simulink model "gm_max_frequency_index"  (R2020a)
settings: Solver=FixedStepDiscrete  StartTime=0.0  StopTime=1e-2  RelTol=1e-3
model workspace (MAT data in the model file):
  amplitud = 2047
  fft_length = 32
  samples_per_period = 3
  sampling_time = 1e-06
libraries: simulink x384, dspsrcs4 x1, dsphdlxfrm x1, dspstat3 x1, hdlsllib x1
(part 15 of 18)

== system gm_max_frequency_index/max_index_frequency/frequency_max/index_finder/for_each_instance30/Iteration6 ==
  xin : Inport  OutDataTypeStr=fixdt(1, 13, 0)  SampleTime=3.2e-05
  yin : Inport  Port=2  OutDataTypeStr=fixdt(1, 13, 0)  SampleTime=3.2e-05
  idx : Inport  Port=3  OutDataTypeStr=fixdt(0, 5, 0)  SampleTime=3.2e-05
  MuxX : Switch  Criteria=u2 ~= 0  Threshold=double(0)  OutDataTypeStr=fixdt(1, 13, 0)  SampleTime=3.2e-05
  MuxY : Switch  Criteria=u2 ~= 0  Threshold=double(0)  OutDataTypeStr=fixdt(1, 13, 0)  SampleTime=3.2e-05
  XAdder : Sum  OutDataTypeStr=fixdt(1, 13, 0)  SampleTime=3.2e-05
  XSubtractor : Sum  Inputs=+-  AccumDataTypeStr=fixdt(1, 13, 0)  OutDataTypeStr=fixdt(1, 13, 0)  SampleTime=3.2e-05
  YAdder : Sum  OutDataTypeStr=fixdt(1, 13, 0)  SampleTime=3.2e-05
  YSub : Sum  Inputs=+-  AccumDataTypeStr=fixdt(1, 13, 0)  OutDataTypeStr=fixdt(1, 13, 0)  SampleTime=3.2e-05
  compare : simulink/Logic and Bit Operations/Compare To Constant  relop=<  const=double(0)  OutDataTypeStr=boolean
  dynamic_shift : ArithShift  BitShiftNumberSource=Input port  BitShiftDirection=Right
      settings: InputPortMap=u0,p1
  dynamic_shift1 : ArithShift  BitShiftNumberSource=Input port  BitShiftDirection=Right
      settings: InputPortMap=u0,p1
  xout : Outport  OutDataTypeStr=fixdt(1, 13, 0)
  yout : Outport  Port=2  OutDataTypeStr=fixdt(1, 13, 0)
  wires:
  idx/1 -> dynamic_shift1/2, dynamic_shift/2
  yin/1 -> YSub/1, YAdder/1, dynamic_shift1/1, compare/1
  xin/1 -> XAdder/1, XSubtractor/1, dynamic_shift/1
  YSub/1 -> MuxY/3
  YAdder/1 -> MuxY/1
  XAdder/1 -> MuxX/3
  XSubtractor/1 -> MuxX/1
  compare/1 -> MuxY/2, MuxX/2
  dynamic_shift1/1 -> XAdder/2, XSubtractor/2
  dynamic_shift/1 -> YSub/2, YAdder/2
  MuxY/1 -> yout/1
  MuxX/1 -> xout/1

== system gm_max_frequency_index/max_index_frequency/frequency_max/index_finder/for_each_instance30/Iteration7 ==
  xin : Inport  OutDataTypeStr=fixdt(1, 13, 0)  SampleTime=3.2e-05
  yin : Inport  Port=2  OutDataTypeStr=fixdt(1, 13, 0)  SampleTime=3.2e-05
  idx : Inport  Port=3  OutDataTypeStr=fixdt(0, 5, 0)  SampleTime=3.2e-05
  MuxX : Switch  Criteria=u2 ~= 0  Threshold=double(0)  OutDataTypeStr=fixdt(1, 13, 0)  SampleTime=3.2e-05
  MuxY : Switch  Criteria=u2 ~= 0  Threshold=double(0)  OutDataTypeStr=fixdt(1, 13, 0)  SampleTime=3.2e-05
  XAdder : Sum  OutDataTypeStr=fixdt(1, 13, 0)  SampleTime=3.2e-05
  XSubtractor : Sum  Inputs=+-  AccumDataTypeStr=fixdt(1, 13, 0)  OutDataTypeStr=fixdt(1, 13, 0)  SampleTime=3.2e-05
  YAdder : Sum  OutDataTypeStr=fixdt(1, 13, 0)  SampleTime=3.2e-05
  YSub : Sum  Inputs=+-  AccumDataTypeStr=fixdt(1, 13, 0)  OutDataTypeStr=fixdt(1, 13, 0)  SampleTime=3.2e-05
  compare : simulink/Logic and Bit Operations/Compare To Constant  relop=<  const=double(0)  OutDataTypeStr=boolean
  dynamic_shift : ArithShift  BitShiftNumberSource=Input port  BitShiftDirection=Right
      settings: InputPortMap=u0,p1
  dynamic_shift1 : ArithShift  BitShiftNumberSource=Input port  BitShiftDirection=Right
      settings: InputPortMap=u0,p1
  xout : Outport  OutDataTypeStr=fixdt(1, 13, 0)
  yout : Outport  Port=2  OutDataTypeStr=fixdt(1, 13, 0)
  wires:
  idx/1 -> dynamic_shift1/2, dynamic_shift/2
  yin/1 -> YSub/1, YAdder/1, dynamic_shift1/1, compare/1
  xin/1 -> XAdder/1, XSubtractor/1, dynamic_shift/1
  YSub/1 -> MuxY/3
  YAdder/1 -> MuxY/1
  XAdder/1 -> MuxX/3
  XSubtractor/1 -> MuxX/1
  compare/1 -> MuxY/2, MuxX/2
  dynamic_shift1/1 -> XAdder/2, XSubtractor/2
  dynamic_shift/1 -> YSub/2, YAdder/2
  MuxY/1 -> yout/1
  MuxX/1 -> xout/1

== system gm_max_frequency_index/max_index_frequency/frequency_max/index_finder/for_each_instance30/Iteration8 ==
  xin : Inport  OutDataTypeStr=fixdt(1, 13, 0)  SampleTime=3.2e-05
  yin : Inport  Port=2  OutDataTypeStr=fixdt(1, 13, 0)  SampleTime=3.2e-05
  idx : Inport  Port=3  OutDataTypeStr=fixdt(0, 5, 0)  SampleTime=3.2e-05
  MuxX : Switch  Criteria=u2 ~= 0  Threshold=double(0)  OutDataTypeStr=fixdt(1, 13, 0)  SampleTime=3.2e-05
  MuxY : Switch  Criteria=u2 ~= 0  Threshold=double(0)  OutDataTypeStr=fixdt(1, 13, 0)  SampleTime=3.2e-05
  XAdder : Sum  OutDataTypeStr=fixdt(1, 13, 0)  SampleTime=3.2e-05
  XSubtractor : Sum  Inputs=+-  AccumDataTypeStr=fixdt(1, 13, 0)  OutDataTypeStr=fixdt(1, 13, 0)  SampleTime=3.2e-05
  YAdder : Sum  OutDataTypeStr=fixdt(1, 13, 0)  SampleTime=3.2e-05
  YSub : Sum  Inputs=+-  AccumDataTypeStr=fixdt(1, 13, 0)  OutDataTypeStr=fixdt(1, 13, 0)  SampleTime=3.2e-05
  compare : simulink/Logic and Bit Operations/Compare To Constant  relop=<  const=double(0)  OutDataTypeStr=boolean
  dynamic_shift : ArithShift  BitShiftNumberSource=Input port  BitShiftDirection=Right
      settings: InputPortMap=u0,p1
  dynamic_shift1 : ArithShift  BitShiftNumberSource=Input port  BitShiftDirection=Right
      settings: InputPortMap=u0,p1
  xout : Outport  OutDataTypeStr=fixdt(1, 13, 0)
  yout : Outport  Port=2  OutDataTypeStr=fixdt(1, 13, 0)
  wires:
  idx/1 -> dynamic_shift1/2, dynamic_shift/2
  yin/1 -> YSub/1, YAdder/1, dynamic_shift1/1, compare/1
  xin/1 -> XAdder/1, XSubtractor/1, dynamic_shift/1
  YSub/1 -> MuxY/3
  YAdder/1 -> MuxY/1
  XAdder/1 -> MuxX/3
  XSubtractor/1 -> MuxX/1
  compare/1 -> MuxY/2, MuxX/2
  dynamic_shift1/1 -> XAdder/2, XSubtractor/2
  dynamic_shift/1 -> YSub/2, YAdder/2
  MuxY/1 -> yout/1
  MuxX/1 -> xout/1

== system gm_max_frequency_index/max_index_frequency/frequency_max/index_finder/for_each_instance30/Iteration9 ==
  xin : Inport  OutDataTypeStr=fixdt(1, 13, 0)  SampleTime=3.2e-05
  yin : Inport  Port=2  OutDataTypeStr=fixdt(1, 13, 0)  SampleTime=3.2e-05
  idx : Inport  Port=3  OutDataTypeStr=fixdt(0, 5, 0)  SampleTime=3.2e-05
  MuxX : Switch  Criteria=u2 ~= 0  Threshold=double(0)  OutDataTypeStr=fixdt(1, 13, 0)  SampleTime=3.2e-05
  MuxY : Switch  Criteria=u2 ~= 0  Threshold=double(0)  OutDataTypeStr=fixdt(1, 13, 0)  SampleTime=3.2e-05
  XAdder : Sum  OutDataTypeStr=fixdt(1, 13, 0)  SampleTime=3.2e-05
  XSubtractor : Sum  Inputs=+-  AccumDataTypeStr=fixdt(1, 13, 0)  OutDataTypeStr=fixdt(1, 13, 0)  SampleTime=3.2e-05
  YAdder : Sum  OutDataTypeStr=fixdt(1, 13, 0)  SampleTime=3.2e-05
  YSub : Sum  Inputs=+-  AccumDataTypeStr=fixdt(1, 13, 0)  OutDataTypeStr=fixdt(1, 13, 0)  SampleTime=3.2e-05
  compare : simulink/Logic and Bit Operations/Compare To Constant  relop=<  const=double(0)  OutDataTypeStr=boolean
  dynamic_shift : ArithShift  BitShiftNumberSource=Input port  BitShiftDirection=Right
      settings: InputPortMap=u0,p1
  dynamic_shift1 : ArithShift  BitShiftNumberSource=Input port  BitShiftDirection=Right
      settings: InputPortMap=u0,p1
  xout : Outport  OutDataTypeStr=fixdt(1, 13, 0)
  yout : Outport  Port=2  OutDataTypeStr=fixdt(1, 13, 0)
  wires:
  idx/1 -> dynamic_shift1/2, dynamic_shift/2
  yin/1 -> YSub/1, YAdder/1, dynamic_shift1/1, compare/1
  xin/1 -> XAdder/1, XSubtractor/1, dynamic_shift/1
  YSub/1 -> MuxY/3
  YAdder/1 -> MuxY/1
  XAdder/1 -> MuxX/3
  XSubtractor/1 -> MuxX/1
  compare/1 -> MuxY/2, MuxX/2
  dynamic_shift1/1 -> XAdder/2, XSubtractor/2
  dynamic_shift/1 -> YSub/2, YAdder/2
  MuxY/1 -> yout/1
  MuxX/1 -> xout/1

== system gm_max_frequency_index/max_index_frequency/frequency_max/index_finder/for_each_instance30/QuadrantMapper ==
  xin : Inport  OutDataTypeStr=fixdt(1, 13, 0)  SampleTime=3.2e-05
  yin : Inport  Port=2  OutDataTypeStr=fixdt(1, 13, 0)  SampleTime=3.2e-05
  abs : Abs  SampleTime=3.2e-05  OutDataTypeStr=fixdt(1, 13, 0)
  abs1 : Abs  SampleTime=3.2e-05  OutDataTypeStr=fixdt(1, 13, 0)
  delayMatch{,1..3} (4 alike) : Delay  DelayLength=double(1)  InitialCondition=0  SampleTime=3.2e-05
  mux : MultiPortSwitch  DataPortOrder=Zero-based contiguous  Inputs=2  DiagnosticForDefault=None  zeroidx=on  OutDataTypeStr=fixdt(1, 13, 0)  SampleTime=3.2e-05
  mux1 : MultiPortSwitch  DataPortOrder=Zero-based contiguous  Inputs=2  DiagnosticForDefault=None  zeroidx=on  OutDataTypeStr=fixdt(1, 13, 0)  SampleTime=3.2e-05
  relop : RelationalOperator  Operator=>  OutDataTypeStr=fixdt(0, 1, 0)  SampleTime=3.2e-05  RndMeth=Nearest  InputSameDT=on
  xout : Outport  OutDataTypeStr=fixdt(1, 13, 0)
  yout : Outport  Port=2  OutDataTypeStr=fixdt(1, 13, 0)
  wires:
  relop/1 -> mux1/1, mux/1
  mux1/1 -> delayMatch3/1
  mux/1 -> delayMatch2/1
  abs1/1 -> delayMatch1/1
  abs/1 -> delayMatch/1
  yin/1 -> abs1/1
  xin/1 -> abs/1
  delayMatch1/1 -> mux/3, mux1/2, relop/2
  delayMatch/1 -> mux/2, mux1/3, relop/1
  delayMatch2/1 -> yout/1
  delayMatch3/1 -> xout/1

== system gm_max_frequency_index/max_index_frequency/frequency_max/index_finder/for_each_instance31/Iteration ==
  xin : Inport  OutDataTypeStr=fixdt(1, 13, 0)  SampleTime=3.2e-05
  yin : Inport  Port=2  OutDataTypeStr=fixdt(1, 13, 0)  SampleTime=3.2e-05
  idx : Inport  Port=3  OutDataTypeStr=fixdt(0, 5, 0)  SampleTime=3.2e-05
  MuxX : Switch  Criteria=u2 ~= 0  Threshold=double(0)  OutDataTypeStr=fixdt(1, 13, 0)  SampleTime=3.2e-05
  MuxY : Switch  Criteria=u2 ~= 0  Threshold=double(0)  OutDataTypeStr=fixdt(1, 13, 0)  SampleTime=3.2e-05
  XAdder : Sum  OutDataTypeStr=fixdt(1, 13, 0)  SampleTime=3.2e-05
  XSubtractor : Sum  Inputs=+-  AccumDataTypeStr=fixdt(1, 13, 0)  OutDataTypeStr=fixdt(1, 13, 0)  SampleTime=3.2e-05
  YAdder : Sum  OutDataTypeStr=fixdt(1, 13, 0)  SampleTime=3.2e-05
  YSub : Sum  Inputs=+-  AccumDataTypeStr=fixdt(1, 13, 0)  OutDataTypeStr=fixdt(1, 13, 0)  SampleTime=3.2e-05
  compare : simulink/Logic and Bit Operations/Compare To Constant  relop=<  const=double(0)  OutDataTypeStr=boolean
  dynamic_shift : ArithShift  BitShiftNumberSource=Input port  BitShiftDirection=Right
      settings: InputPortMap=u0,p1
  dynamic_shift1 : ArithShift  BitShiftNumberSource=Input port  BitShiftDirection=Right
      settings: InputPortMap=u0,p1
  xout : Outport  OutDataTypeStr=fixdt(1, 13, 0)
  yout : Outport  Port=2  OutDataTypeStr=fixdt(1, 13, 0)
  wires:
  idx/1 -> dynamic_shift1/2, dynamic_shift/2
  yin/1 -> YSub/1, YAdder/1, dynamic_shift1/1, compare/1
  xin/1 -> XAdder/1, XSubtractor/1, dynamic_shift/1
  YSub/1 -> MuxY/3
  YAdder/1 -> MuxY/1
  XAdder/1 -> MuxX/3
  XSubtractor/1 -> MuxX/1
  compare/1 -> MuxY/2, MuxX/2
  dynamic_shift1/1 -> XAdder/2, XSubtractor/2
  dynamic_shift/1 -> YSub/2, YAdder/2
  MuxY/1 -> yout/1
  MuxX/1 -> xout/1

== system gm_max_frequency_index/max_index_frequency/frequency_max/index_finder/for_each_instance31/Iteration1 ==
  xin : Inport  OutDataTypeStr=fixdt(1, 13, 0)  SampleTime=3.2e-05
  yin : Inport  Port=2  OutDataTypeStr=fixdt(1, 13, 0)  SampleTime=3.2e-05
  idx : Inport  Port=3  OutDataTypeStr=fixdt(0, 5, 0)  SampleTime=3.2e-05
  MuxX : Switch  Criteria=u2 ~= 0  Threshold=double(0)  OutDataTypeStr=fixdt(1, 13, 0)  SampleTime=3.2e-05
  MuxY : Switch  Criteria=u2 ~= 0  Threshold=double(0)  OutDataTypeStr=fixdt(1, 13, 0)  SampleTime=3.2e-05
  XAdder : Sum  OutDataTypeStr=fixdt(1, 13, 0)  SampleTime=3.2e-05
  XSubtractor : Sum  Inputs=+-  AccumDataTypeStr=fixdt(1, 13, 0)  OutDataTypeStr=fixdt(1, 13, 0)  SampleTime=3.2e-05
  YAdder : Sum  OutDataTypeStr=fixdt(1, 13, 0)  SampleTime=3.2e-05
  YSub : Sum  Inputs=+-  AccumDataTypeStr=fixdt(1, 13, 0)  OutDataTypeStr=fixdt(1, 13, 0)  SampleTime=3.2e-05
  compare : simulink/Logic and Bit Operations/Compare To Constant  relop=<  const=double(0)  OutDataTypeStr=boolean
  dynamic_shift : ArithShift  BitShiftNumberSource=Input port  BitShiftDirection=Right
      settings: InputPortMap=u0,p1
  dynamic_shift1 : ArithShift  BitShiftNumberSource=Input port  BitShiftDirection=Right
      settings: InputPortMap=u0,p1
  xout : Outport  OutDataTypeStr=fixdt(1, 13, 0)
  yout : Outport  Port=2  OutDataTypeStr=fixdt(1, 13, 0)
  wires:
  idx/1 -> dynamic_shift1/2, dynamic_shift/2
  yin/1 -> YSub/1, YAdder/1, dynamic_shift1/1, compare/1
  xin/1 -> XAdder/1, XSubtractor/1, dynamic_shift/1
  YSub/1 -> MuxY/3
  YAdder/1 -> MuxY/1
  XAdder/1 -> MuxX/3
  XSubtractor/1 -> MuxX/1
  compare/1 -> MuxY/2, MuxX/2
  dynamic_shift1/1 -> XAdder/2, XSubtractor/2
  dynamic_shift/1 -> YSub/2, YAdder/2
  MuxY/1 -> yout/1
  MuxX/1 -> xout/1

== system gm_max_frequency_index/max_index_frequency/frequency_max/index_finder/for_each_instance31/Iteration10 ==
  xin : Inport  OutDataTypeStr=fixdt(1, 13, 0)  SampleTime=3.2e-05
  yin : Inport  Port=2  OutDataTypeStr=fixdt(1, 13, 0)  SampleTime=3.2e-05
  idx : Inport  Port=3  OutDataTypeStr=fixdt(0, 5, 0)  SampleTime=3.2e-05
  MuxX : Switch  Criteria=u2 ~= 0  Threshold=double(0)  OutDataTypeStr=fixdt(1, 13, 0)  SampleTime=3.2e-05
  MuxY : Switch  Criteria=u2 ~= 0  Threshold=double(0)  OutDataTypeStr=fixdt(1, 13, 0)  SampleTime=3.2e-05
  XAdder : Sum  OutDataTypeStr=fixdt(1, 13, 0)  SampleTime=3.2e-05
  XSubtractor : Sum  Inputs=+-  AccumDataTypeStr=fixdt(1, 13, 0)  OutDataTypeStr=fixdt(1, 13, 0)  SampleTime=3.2e-05
  YAdder : Sum  OutDataTypeStr=fixdt(1, 13, 0)  SampleTime=3.2e-05
  YSub : Sum  Inputs=+-  AccumDataTypeStr=fixdt(1, 13, 0)  OutDataTypeStr=fixdt(1, 13, 0)  SampleTime=3.2e-05
  compare : simulink/Logic and Bit Operations/Compare To Constant  relop=<  const=double(0)  OutDataTypeStr=boolean
  dynamic_shift : ArithShift  BitShiftNumberSource=Input port  BitShiftDirection=Right
      settings: InputPortMap=u0,p1
  dynamic_shift1 : ArithShift  BitShiftNumberSource=Input port  BitShiftDirection=Right
      settings: InputPortMap=u0,p1
  xout : Outport  OutDataTypeStr=fixdt(1, 13, 0)
  yout : Outport  Port=2  OutDataTypeStr=fixdt(1, 13, 0)
  wires:
  idx/1 -> dynamic_shift/2, dynamic_shift1/2
  yin/1 -> compare/1, dynamic_shift1/1, YAdder/1, YSub/1
  xin/1 -> dynamic_shift/1, XSubtractor/1, XAdder/1
  YSub/1 -> MuxY/3
  YAdder/1 -> MuxY/1
  XAdder/1 -> MuxX/3
  XSubtractor/1 -> MuxX/1
  compare/1 -> MuxX/2, MuxY/2
  dynamic_shift1/1 -> XSubtractor/2, XAdder/2
  dynamic_shift/1 -> YAdder/2, YSub/2
  MuxY/1 -> yout/1
  MuxX/1 -> xout/1

== system gm_max_frequency_index/max_index_frequency/frequency_max/index_finder/for_each_instance31/Iteration2 ==
  xin : Inport  OutDataTypeStr=fixdt(1, 13, 0)  SampleTime=3.2e-05
  yin : Inport  Port=2  OutDataTypeStr=fixdt(1, 13, 0)  SampleTime=3.2e-05
  idx : Inport  Port=3  OutDataTypeStr=fixdt(0, 5, 0)  SampleTime=3.2e-05
  MuxX : Switch  Criteria=u2 ~= 0  Threshold=double(0)  OutDataTypeStr=fixdt(1, 13, 0)  SampleTime=3.2e-05
  MuxY : Switch  Criteria=u2 ~= 0  Threshold=double(0)  OutDataTypeStr=fixdt(1, 13, 0)  SampleTime=3.2e-05
  XAdder : Sum  OutDataTypeStr=fixdt(1, 13, 0)  SampleTime=3.2e-05
  XSubtractor : Sum  Inputs=+-  AccumDataTypeStr=fixdt(1, 13, 0)  OutDataTypeStr=fixdt(1, 13, 0)  SampleTime=3.2e-05
  YAdder : Sum  OutDataTypeStr=fixdt(1, 13, 0)  SampleTime=3.2e-05
  YSub : Sum  Inputs=+-  AccumDataTypeStr=fixdt(1, 13, 0)  OutDataTypeStr=fixdt(1, 13, 0)  SampleTime=3.2e-05
  compare : simulink/Logic and Bit Operations/Compare To Constant  relop=<  const=double(0)  OutDataTypeStr=boolean
  dynamic_shift : ArithShift  BitShiftNumberSource=Input port  BitShiftDirection=Right
      settings: InputPortMap=u0,p1
  dynamic_shift1 : ArithShift  BitShiftNumberSource=Input port  BitShiftDirection=Right
      settings: InputPortMap=u0,p1
  xout : Outport  OutDataTypeStr=fixdt(1, 13, 0)
  yout : Outport  Port=2  OutDataTypeStr=fixdt(1, 13, 0)
  wires:
  idx/1 -> dynamic_shift1/2, dynamic_shift/2
  yin/1 -> YSub/1, YAdder/1, dynamic_shift1/1, compare/1
  xin/1 -> XAdder/1, XSubtractor/1, dynamic_shift/1
  YSub/1 -> MuxY/3
  YAdder/1 -> MuxY/1
  XAdder/1 -> MuxX/3
  XSubtractor/1 -> MuxX/1
  compare/1 -> MuxY/2, MuxX/2
  dynamic_shift1/1 -> XAdder/2, XSubtractor/2
  dynamic_shift/1 -> YSub/2, YAdder/2
  MuxY/1 -> yout/1
  MuxX/1 -> xout/1

== system gm_max_frequency_index/max_index_frequency/frequency_max/index_finder/for_each_instance31/Iteration3 ==
  xin : Inport  OutDataTypeStr=fixdt(1, 13, 0)  SampleTime=3.2e-05
  yin : Inport  Port=2  OutDataTypeStr=fixdt(1, 13, 0)  SampleTime=3.2e-05
  idx : Inport  Port=3  OutDataTypeStr=fixdt(0, 5, 0)  SampleTime=3.2e-05
  MuxX : Switch  Criteria=u2 ~= 0  Threshold=double(0)  OutDataTypeStr=fixdt(1, 13, 0)  SampleTime=3.2e-05
  MuxY : Switch  Criteria=u2 ~= 0  Threshold=double(0)  OutDataTypeStr=fixdt(1, 13, 0)  SampleTime=3.2e-05
  XAdder : Sum  OutDataTypeStr=fixdt(1, 13, 0)  SampleTime=3.2e-05
  XSubtractor : Sum  Inputs=+-  AccumDataTypeStr=fixdt(1, 13, 0)  OutDataTypeStr=fixdt(1, 13, 0)  SampleTime=3.2e-05
  YAdder : Sum  OutDataTypeStr=fixdt(1, 13, 0)  SampleTime=3.2e-05
  YSub : Sum  Inputs=+-  AccumDataTypeStr=fixdt(1, 13, 0)  OutDataTypeStr=fixdt(1, 13, 0)  SampleTime=3.2e-05
  compare : simulink/Logic and Bit Operations/Compare To Constant  relop=<  const=double(0)  OutDataTypeStr=boolean
  dynamic_shift : ArithShift  BitShiftNumberSource=Input port  BitShiftDirection=Right
      settings: InputPortMap=u0,p1
  dynamic_shift1 : ArithShift  BitShiftNumberSource=Input port  BitShiftDirection=Right
      settings: InputPortMap=u0,p1
  xout : Outport  OutDataTypeStr=fixdt(1, 13, 0)
  yout : Outport  Port=2  OutDataTypeStr=fixdt(1, 13, 0)
  wires:
  idx/1 -> dynamic_shift1/2, dynamic_shift/2
  yin/1 -> YSub/1, YAdder/1, dynamic_shift1/1, compare/1
  xin/1 -> XAdder/1, XSubtractor/1, dynamic_shift/1
  YSub/1 -> MuxY/3
  YAdder/1 -> MuxY/1
  XAdder/1 -> MuxX/3
  XSubtractor/1 -> MuxX/1
  compare/1 -> MuxY/2, MuxX/2
  dynamic_shift1/1 -> XAdder/2, XSubtractor/2
  dynamic_shift/1 -> YSub/2, YAdder/2
  MuxY/1 -> yout/1
  MuxX/1 -> xout/1

== system gm_max_frequency_index/max_index_frequency/frequency_max/index_finder/for_each_instance31/Iteration4 ==
  xin : Inport  OutDataTypeStr=fixdt(1, 13, 0)  SampleTime=3.2e-05
  yin : Inport  Port=2  OutDataTypeStr=fixdt(1, 13, 0)  SampleTime=3.2e-05
  idx : Inport  Port=3  OutDataTypeStr=fixdt(0, 5, 0)  SampleTime=3.2e-05
  MuxX : Switch  Criteria=u2 ~= 0  Threshold=double(0)  OutDataTypeStr=fixdt(1, 13, 0)  SampleTime=3.2e-05
  MuxY : Switch  Criteria=u2 ~= 0  Threshold=double(0)  OutDataTypeStr=fixdt(1, 13, 0)  SampleTime=3.2e-05
  XAdder : Sum  OutDataTypeStr=fixdt(1, 13, 0)  SampleTime=3.2e-05
  XSubtractor : Sum  Inputs=+-  AccumDataTypeStr=fixdt(1, 13, 0)  OutDataTypeStr=fixdt(1, 13, 0)  SampleTime=3.2e-05
  YAdder : Sum  OutDataTypeStr=fixdt(1, 13, 0)  SampleTime=3.2e-05
  YSub : Sum  Inputs=+-  AccumDataTypeStr=fixdt(1, 13, 0)  OutDataTypeStr=fixdt(1, 13, 0)  SampleTime=3.2e-05
  compare : simulink/Logic and Bit Operations/Compare To Constant  relop=<  const=double(0)  OutDataTypeStr=boolean
  dynamic_shift : ArithShift  BitShiftNumberSource=Input port  BitShiftDirection=Right
      settings: InputPortMap=u0,p1
  dynamic_shift1 : ArithShift  BitShiftNumberSource=Input port  BitShiftDirection=Right
      settings: InputPortMap=u0,p1
  xout : Outport  OutDataTypeStr=fixdt(1, 13, 0)
  yout : Outport  Port=2  OutDataTypeStr=fixdt(1, 13, 0)
  wires:
  idx/1 -> dynamic_shift1/2, dynamic_shift/2
  yin/1 -> YSub/1, YAdder/1, dynamic_shift1/1, compare/1
  xin/1 -> XAdder/1, XSubtractor/1, dynamic_shift/1
  YSub/1 -> MuxY/3
  YAdder/1 -> MuxY/1
  XAdder/1 -> MuxX/3
  XSubtractor/1 -> MuxX/1
  compare/1 -> MuxY/2, MuxX/2
  dynamic_shift1/1 -> XAdder/2, XSubtractor/2
  dynamic_shift/1 -> YSub/2, YAdder/2
  MuxY/1 -> yout/1
  MuxX/1 -> xout/1

== system gm_max_frequency_index/max_index_frequency/frequency_max/index_finder/for_each_instance31/Iteration5 ==
  xin : Inport  OutDataTypeStr=fixdt(1, 13, 0)  SampleTime=3.2e-05
  yin : Inport  Port=2  OutDataTypeStr=fixdt(1, 13, 0)  SampleTime=3.2e-05
  idx : Inport  Port=3  OutDataTypeStr=fixdt(0, 5, 0)  SampleTime=3.2e-05
  MuxX : Switch  Criteria=u2 ~= 0  Threshold=double(0)  OutDataTypeStr=fixdt(1, 13, 0)  SampleTime=3.2e-05
  MuxY : Switch  Criteria=u2 ~= 0  Threshold=double(0)  OutDataTypeStr=fixdt(1, 13, 0)  SampleTime=3.2e-05
  XAdder : Sum  OutDataTypeStr=fixdt(1, 13, 0)  SampleTime=3.2e-05
  XSubtractor : Sum  Inputs=+-  AccumDataTypeStr=fixdt(1, 13, 0)  OutDataTypeStr=fixdt(1, 13, 0)  SampleTime=3.2e-05
  YAdder : Sum  OutDataTypeStr=fixdt(1, 13, 0)  SampleTime=3.2e-05
  YSub : Sum  Inputs=+-  AccumDataTypeStr=fixdt(1, 13, 0)  OutDataTypeStr=fixdt(1, 13, 0)  SampleTime=3.2e-05
  compare : simulink/Logic and Bit Operations/Compare To Constant  relop=<  const=double(0)  OutDataTypeStr=boolean
  dynamic_shift : ArithShift  BitShiftNumberSource=Input port  BitShiftDirection=Right
      settings: InputPortMap=u0,p1
  dynamic_shift1 : ArithShift  BitShiftNumberSource=Input port  BitShiftDirection=Right
      settings: InputPortMap=u0,p1
  xout : Outport  OutDataTypeStr=fixdt(1, 13, 0)
  yout : Outport  Port=2  OutDataTypeStr=fixdt(1, 13, 0)
  wires:
  idx/1 -> dynamic_shift1/2, dynamic_shift/2
  yin/1 -> YSub/1, YAdder/1, dynamic_shift1/1, compare/1
  xin/1 -> XAdder/1, XSubtractor/1, dynamic_shift/1
  YSub/1 -> MuxY/3
  YAdder/1 -> MuxY/1
  XAdder/1 -> MuxX/3
  XSubtractor/1 -> MuxX/1
  compare/1 -> MuxY/2, MuxX/2
  dynamic_shift1/1 -> XAdder/2, XSubtractor/2
  dynamic_shift/1 -> YSub/2, YAdder/2
  MuxY/1 -> yout/1
  MuxX/1 -> xout/1

== system gm_max_frequency_index/max_index_frequency/frequency_max/index_finder/for_each_instance31/Iteration6 ==
  xin : Inport  OutDataTypeStr=fixdt(1, 13, 0)  SampleTime=3.2e-05
  yin : Inport  Port=2  OutDataTypeStr=fixdt(1, 13, 0)  SampleTime=3.2e-05
  idx : Inport  Port=3  OutDataTypeStr=fixdt(0, 5, 0)  SampleTime=3.2e-05
  MuxX : Switch  Criteria=u2 ~= 0  Threshold=double(0)  OutDataTypeStr=fixdt(1, 13, 0)  SampleTime=3.2e-05
  MuxY : Switch  Criteria=u2 ~= 0  Threshold=double(0)  OutDataTypeStr=fixdt(1, 13, 0)  SampleTime=3.2e-05
  XAdder : Sum  OutDataTypeStr=fixdt(1, 13, 0)  SampleTime=3.2e-05
  XSubtractor : Sum  Inputs=+-  AccumDataTypeStr=fixdt(1, 13, 0)  OutDataTypeStr=fixdt(1, 13, 0)  SampleTime=3.2e-05
  YAdder : Sum  OutDataTypeStr=fixdt(1, 13, 0)  SampleTime=3.2e-05
  YSub : Sum  Inputs=+-  AccumDataTypeStr=fixdt(1, 13, 0)  OutDataTypeStr=fixdt(1, 13, 0)  SampleTime=3.2e-05
  compare : simulink/Logic and Bit Operations/Compare To Constant  relop=<  const=double(0)  OutDataTypeStr=boolean
  dynamic_shift : ArithShift  BitShiftNumberSource=Input port  BitShiftDirection=Right
      settings: InputPortMap=u0,p1
  dynamic_shift1 : ArithShift  BitShiftNumberSource=Input port  BitShiftDirection=Right
      settings: InputPortMap=u0,p1
  xout : Outport  OutDataTypeStr=fixdt(1, 13, 0)
  yout : Outport  Port=2  OutDataTypeStr=fixdt(1, 13, 0)
  wires:
  idx/1 -> dynamic_shift1/2, dynamic_shift/2
  yin/1 -> YSub/1, YAdder/1, dynamic_shift1/1, compare/1
  xin/1 -> XAdder/1, XSubtractor/1, dynamic_shift/1
  YSub/1 -> MuxY/3
  YAdder/1 -> MuxY/1
  XAdder/1 -> MuxX/3
  XSubtractor/1 -> MuxX/1
  compare/1 -> MuxY/2, MuxX/2
  dynamic_shift1/1 -> XAdder/2, XSubtractor/2
  dynamic_shift/1 -> YSub/2, YAdder/2
  MuxY/1 -> yout/1
  MuxX/1 -> xout/1

== system gm_max_frequency_index/max_index_frequency/frequency_max/index_finder/for_each_instance31/Iteration7 ==
  xin : Inport  OutDataTypeStr=fixdt(1, 13, 0)  SampleTime=3.2e-05
  yin : Inport  Port=2  OutDataTypeStr=fixdt(1, 13, 0)  SampleTime=3.2e-05
  idx : Inport  Port=3  OutDataTypeStr=fixdt(0, 5, 0)  SampleTime=3.2e-05
  MuxX : Switch  Criteria=u2 ~= 0  Threshold=double(0)  OutDataTypeStr=fixdt(1, 13, 0)  SampleTime=3.2e-05
  MuxY : Switch  Criteria=u2 ~= 0  Threshold=double(0)  OutDataTypeStr=fixdt(1, 13, 0)  SampleTime=3.2e-05
  XAdder : Sum  OutDataTypeStr=fixdt(1, 13, 0)  SampleTime=3.2e-05
  XSubtractor : Sum  Inputs=+-  AccumDataTypeStr=fixdt(1, 13, 0)  OutDataTypeStr=fixdt(1, 13, 0)  SampleTime=3.2e-05
  YAdder : Sum  OutDataTypeStr=fixdt(1, 13, 0)  SampleTime=3.2e-05
  YSub : Sum  Inputs=+-  AccumDataTypeStr=fixdt(1, 13, 0)  OutDataTypeStr=fixdt(1, 13, 0)  SampleTime=3.2e-05
  compare : simulink/Logic and Bit Operations/Compare To Constant  relop=<  const=double(0)  OutDataTypeStr=boolean
  dynamic_shift : ArithShift  BitShiftNumberSource=Input port  BitShiftDirection=Right
      settings: InputPortMap=u0,p1
  dynamic_shift1 : ArithShift  BitShiftNumberSource=Input port  BitShiftDirection=Right
      settings: InputPortMap=u0,p1
  xout : Outport  OutDataTypeStr=fixdt(1, 13, 0)
  yout : Outport  Port=2  OutDataTypeStr=fixdt(1, 13, 0)
  wires:
  idx/1 -> dynamic_shift1/2, dynamic_shift/2
  yin/1 -> YSub/1, YAdder/1, dynamic_shift1/1, compare/1
  xin/1 -> XAdder/1, XSubtractor/1, dynamic_shift/1
  YSub/1 -> MuxY/3
  YAdder/1 -> MuxY/1
  XAdder/1 -> MuxX/3
  XSubtractor/1 -> MuxX/1
  compare/1 -> MuxY/2, MuxX/2
  dynamic_shift1/1 -> XAdder/2, XSubtractor/2
  dynamic_shift/1 -> YSub/2, YAdder/2
  MuxY/1 -> yout/1
  MuxX/1 -> xout/1

== system gm_max_frequency_index/max_index_frequency/frequency_max/index_finder/for_each_instance31/Iteration8 ==
  xin : Inport  OutDataTypeStr=fixdt(1, 13, 0)  SampleTime=3.2e-05
  yin : Inport  Port=2  OutDataTypeStr=fixdt(1, 13, 0)  SampleTime=3.2e-05
  idx : Inport  Port=3  OutDataTypeStr=fixdt(0, 5, 0)  SampleTime=3.2e-05
  MuxX : Switch  Criteria=u2 ~= 0  Threshold=double(0)  OutDataTypeStr=fixdt(1, 13, 0)  SampleTime=3.2e-05
  MuxY : Switch  Criteria=u2 ~= 0  Threshold=double(0)  OutDataTypeStr=fixdt(1, 13, 0)  SampleTime=3.2e-05
  XAdder : Sum  OutDataTypeStr=fixdt(1, 13, 0)  SampleTime=3.2e-05
  XSubtractor : Sum  Inputs=+-  AccumDataTypeStr=fixdt(1, 13, 0)  OutDataTypeStr=fixdt(1, 13, 0)  SampleTime=3.2e-05
  YAdder : Sum  OutDataTypeStr=fixdt(1, 13, 0)  SampleTime=3.2e-05
  YSub : Sum  Inputs=+-  AccumDataTypeStr=fixdt(1, 13, 0)  OutDataTypeStr=fixdt(1, 13, 0)  SampleTime=3.2e-05
  compare : simulink/Logic and Bit Operations/Compare To Constant  relop=<  const=double(0)  OutDataTypeStr=boolean
  dynamic_shift : ArithShift  BitShiftNumberSource=Input port  BitShiftDirection=Right
      settings: InputPortMap=u0,p1
  dynamic_shift1 : ArithShift  BitShiftNumberSource=Input port  BitShiftDirection=Right
      settings: InputPortMap=u0,p1
  xout : Outport  OutDataTypeStr=fixdt(1, 13, 0)
  yout : Outport  Port=2  OutDataTypeStr=fixdt(1, 13, 0)
  wires:
  idx/1 -> dynamic_shift1/2, dynamic_shift/2
  yin/1 -> YSub/1, YAdder/1, dynamic_shift1/1, compare/1
  xin/1 -> XAdder/1, XSubtractor/1, dynamic_shift/1
  YSub/1 -> MuxY/3
  YAdder/1 -> MuxY/1
  XAdder/1 -> MuxX/3
  XSubtractor/1 -> MuxX/1
  compare/1 -> MuxY/2, MuxX/2
  dynamic_shift1/1 -> XAdder/2, XSubtractor/2
  dynamic_shift/1 -> YSub/2, YAdder/2
  MuxY/1 -> yout/1
  MuxX/1 -> xout/1

== system gm_max_frequency_index/max_index_frequency/frequency_max/index_finder/for_each_instance31/Iteration9 ==
  xin : Inport  OutDataTypeStr=fixdt(1, 13, 0)  SampleTime=3.2e-05
  yin : Inport  Port=2  OutDataTypeStr=fixdt(1, 13, 0)  SampleTime=3.2e-05
  idx : Inport  Port=3  OutDataTypeStr=fixdt(0, 5, 0)  SampleTime=3.2e-05
  MuxX : Switch  Criteria=u2 ~= 0  Threshold=double(0)  OutDataTypeStr=fixdt(1, 13, 0)  SampleTime=3.2e-05
  MuxY : Switch  Criteria=u2 ~= 0  Threshold=double(0)  OutDataTypeStr=fixdt(1, 13, 0)  SampleTime=3.2e-05
  XAdder : Sum  OutDataTypeStr=fixdt(1, 13, 0)  SampleTime=3.2e-05
  XSubtractor : Sum  Inputs=+-  AccumDataTypeStr=fixdt(1, 13, 0)  OutDataTypeStr=fixdt(1, 13, 0)  SampleTime=3.2e-05
  YAdder : Sum  OutDataTypeStr=fixdt(1, 13, 0)  SampleTime=3.2e-05
  YSub : Sum  Inputs=+-  AccumDataTypeStr=fixdt(1, 13, 0)  OutDataTypeStr=fixdt(1, 13, 0)  SampleTime=3.2e-05
  compare : simulink/Logic and Bit Operations/Compare To Constant  relop=<  const=double(0)  OutDataTypeStr=boolean
  dynamic_shift : ArithShift  BitShiftNumberSource=Input port  BitShiftDirection=Right
      settings: InputPortMap=u0,p1
  dynamic_shift1 : ArithShift  BitShiftNumberSource=Input port  BitShiftDirection=Right
      settings: InputPortMap=u0,p1
  xout : Outport  OutDataTypeStr=fixdt(1, 13, 0)
  yout : Outport  Port=2  OutDataTypeStr=fixdt(1, 13, 0)
  wires:
  idx/1 -> dynamic_shift1/2, dynamic_shift/2
  yin/1 -> YSub/1, YAdder/1, dynamic_shift1/1, compare/1
  xin/1 -> XAdder/1, XSubtractor/1, dynamic_shift/1
  YSub/1 -> MuxY/3
  YAdder/1 -> MuxY/1
  XAdder/1 -> MuxX/3
  XSubtractor/1 -> MuxX/1
  compare/1 -> MuxY/2, MuxX/2
  dynamic_shift1/1 -> XAdder/2, XSubtractor/2
  dynamic_shift/1 -> YSub/2, YAdder/2
  MuxY/1 -> yout/1
  MuxX/1 -> xout/1

== system gm_max_frequency_index/max_index_frequency/frequency_max/index_finder/for_each_instance31/QuadrantMapper ==
  xin : Inport  OutDataTypeStr=fixdt(1, 13, 0)  SampleTime=3.2e-05
  yin : Inport  Port=2  OutDataTypeStr=fixdt(1, 13, 0)  SampleTime=3.2e-05
  abs : Abs  SampleTime=3.2e-05  OutDataTypeStr=fixdt(1, 13, 0)
  abs1 : Abs  SampleTime=3.2e-05  OutDataTypeStr=fixdt(1, 13, 0)
  delayMatch{,1..3} (4 alike) : Delay  DelayLength=double(1)  InitialCondition=0  SampleTime=3.2e-05
  mux : MultiPortSwitch  DataPortOrder=Zero-based contiguous  Inputs=2  DiagnosticForDefault=None  zeroidx=on  OutDataTypeStr=fixdt(1, 13, 0)  SampleTime=3.2e-05
  mux1 : MultiPortSwitch  DataPortOrder=Zero-based contiguous  Inputs=2  DiagnosticForDefault=None  zeroidx=on  OutDataTypeStr=fixdt(1, 13, 0)  SampleTime=3.2e-05
  relop : RelationalOperator  Operator=>  OutDataTypeStr=fixdt(0, 1, 0)  SampleTime=3.2e-05  RndMeth=Nearest  InputSameDT=on
  xout : Outport  OutDataTypeStr=fixdt(1, 13, 0)
  yout : Outport  Port=2  OutDataTypeStr=fixdt(1, 13, 0)
  wires:
  relop/1 -> mux1/1, mux/1
  mux1/1 -> delayMatch3/1
  mux/1 -> delayMatch2/1
  abs1/1 -> delayMatch1/1
  abs/1 -> delayMatch/1
  yin/1 -> abs1/1
  xin/1 -> abs/1
  delayMatch1/1 -> mux/3, mux1/2, relop/2
  delayMatch/1 -> mux/2, mux1/3, relop/1
  delayMatch2/1 -> yout/1
  delayMatch3/1 -> xout/1

== system gm_max_frequency_index/max_index_frequency/frequency_max/index_finder/for_each_instance32/Iteration ==
  xin : Inport  OutDataTypeStr=fixdt(1, 13, 0)  SampleTime=3.2e-05
  yin : Inport  Port=2  OutDataTypeStr=fixdt(1, 13, 0)  SampleTime=3.2e-05
  idx : Inport  Port=3  OutDataTypeStr=fixdt(0, 5, 0)  SampleTime=3.2e-05
  MuxX : Switch  Criteria=u2 ~= 0  Threshold=double(0)  OutDataTypeStr=fixdt(1, 13, 0)  SampleTime=3.2e-05
  MuxY : Switch  Criteria=u2 ~= 0  Threshold=double(0)  OutDataTypeStr=fixdt(1, 13, 0)  SampleTime=3.2e-05
  XAdder : Sum  OutDataTypeStr=fixdt(1, 13, 0)  SampleTime=3.2e-05
  XSubtractor : Sum  Inputs=+-  AccumDataTypeStr=fixdt(1, 13, 0)  OutDataTypeStr=fixdt(1, 13, 0)  SampleTime=3.2e-05
  YAdder : Sum  OutDataTypeStr=fixdt(1, 13, 0)  SampleTime=3.2e-05
  YSub : Sum  Inputs=+-  AccumDataTypeStr=fixdt(1, 13, 0)  OutDataTypeStr=fixdt(1, 13, 0)  SampleTime=3.2e-05
  compare : simulink/Logic and Bit Operations/Compare To Constant  relop=<  const=double(0)  OutDataTypeStr=boolean
  dynamic_shift : ArithShift  BitShiftNumberSource=Input port  BitShiftDirection=Right
      settings: InputPortMap=u0,p1
  dynamic_shift1 : ArithShift  BitShiftNumberSource=Input port  BitShiftDirection=Right
      settings: InputPortMap=u0,p1
  xout : Outport  OutDataTypeStr=fixdt(1, 13, 0)
  yout : Outport  Port=2  OutDataTypeStr=fixdt(1, 13, 0)
  wires:
  idx/1 -> dynamic_shift1/2, dynamic_shift/2
  yin/1 -> YSub/1, YAdder/1, dynamic_shift1/1, compare/1
  xin/1 -> XAdder/1, XSubtractor/1, dynamic_shift/1
  YSub/1 -> MuxY/3
  YAdder/1 -> MuxY/1
  XAdder/1 -> MuxX/3
  XSubtractor/1 -> MuxX/1
  compare/1 -> MuxY/2, MuxX/2
  dynamic_shift1/1 -> XAdder/2, XSubtractor/2
  dynamic_shift/1 -> YSub/2, YAdder/2
  MuxY/1 -> yout/1
  MuxX/1 -> xout/1

== system gm_max_frequency_index/max_index_frequency/frequency_max/index_finder/for_each_instance32/Iteration1 ==
  xin : Inport  OutDataTypeStr=fixdt(1, 13, 0)  SampleTime=3.2e-05
  yin : Inport  Port=2  OutDataTypeStr=fixdt(1, 13, 0)  SampleTime=3.2e-05
  idx : Inport  Port=3  OutDataTypeStr=fixdt(0, 5, 0)  SampleTime=3.2e-05
  MuxX : Switch  Criteria=u2 ~= 0  Threshold=double(0)  OutDataTypeStr=fixdt(1, 13, 0)  SampleTime=3.2e-05
  MuxY : Switch  Criteria=u2 ~= 0  Threshold=double(0)  OutDataTypeStr=fixdt(1, 13, 0)  SampleTime=3.2e-05
  XAdder : Sum  OutDataTypeStr=fixdt(1, 13, 0)  SampleTime=3.2e-05
  XSubtractor : Sum  Inputs=+-  AccumDataTypeStr=fixdt(1, 13, 0)  OutDataTypeStr=fixdt(1, 13, 0)  SampleTime=3.2e-05
  YAdder : Sum  OutDataTypeStr=fixdt(1, 13, 0)  SampleTime=3.2e-05
  YSub : Sum  Inputs=+-  AccumDataTypeStr=fixdt(1, 13, 0)  OutDataTypeStr=fixdt(1, 13, 0)  SampleTime=3.2e-05
  compare : simulink/Logic and Bit Operations/Compare To Constant  relop=<  const=double(0)  OutDataTypeStr=boolean
  dynamic_shift : ArithShift  BitShiftNumberSource=Input port  BitShiftDirection=Right
      settings: InputPortMap=u0,p1
  dynamic_shift1 : ArithShift  BitShiftNumberSource=Input port  BitShiftDirection=Right
      settings: InputPortMap=u0,p1
  xout : Outport  OutDataTypeStr=fixdt(1, 13, 0)
  yout : Outport  Port=2  OutDataTypeStr=fixdt(1, 13, 0)
  wires:
  idx/1 -> dynamic_shift1/2, dynamic_shift/2
  yin/1 -> YSub/1, YAdder/1, dynamic_shift1/1, compare/1
  xin/1 -> XAdder/1, XSubtractor/1, dynamic_shift/1
  YSub/1 -> MuxY/3
  YAdder/1 -> MuxY/1
  XAdder/1 -> MuxX/3
  XSubtractor/1 -> MuxX/1
  compare/1 -> MuxY/2, MuxX/2
  dynamic_shift1/1 -> XAdder/2, XSubtractor/2
  dynamic_shift/1 -> YSub/2, YAdder/2
  MuxY/1 -> yout/1
  MuxX/1 -> xout/1

== system gm_max_frequency_index/max_index_frequency/frequency_max/index_finder/for_each_instance32/Iteration10 ==
  xin : Inport  OutDataTypeStr=fixdt(1, 13, 0)  SampleTime=3.2e-05
  yin : Inport  Port=2  OutDataTypeStr=fixdt(1, 13, 0)  SampleTime=3.2e-05
  idx : Inport  Port=3  OutDataTypeStr=fixdt(0, 5, 0)  SampleTime=3.2e-05
  MuxX : Switch  Criteria=u2 ~= 0  Threshold=double(0)  OutDataTypeStr=fixdt(1, 13, 0)  SampleTime=3.2e-05
  MuxY : Switch  Criteria=u2 ~= 0  Threshold=double(0)  OutDataTypeStr=fixdt(1, 13, 0)  SampleTime=3.2e-05
  XAdder : Sum  OutDataTypeStr=fixdt(1, 13, 0)  SampleTime=3.2e-05
  XSubtractor : Sum  Inputs=+-  AccumDataTypeStr=fixdt(1, 13, 0)  OutDataTypeStr=fixdt(1, 13, 0)  SampleTime=3.2e-05
  YAdder : Sum  OutDataTypeStr=fixdt(1, 13, 0)  SampleTime=3.2e-05
  YSub : Sum  Inputs=+-  AccumDataTypeStr=fixdt(1, 13, 0)  OutDataTypeStr=fixdt(1, 13, 0)  SampleTime=3.2e-05
  compare : simulink/Logic and Bit Operations/Compare To Constant  relop=<  const=double(0)  OutDataTypeStr=boolean
  dynamic_shift : ArithShift  BitShiftNumberSource=Input port  BitShiftDirection=Right
      settings: InputPortMap=u0,p1
  dynamic_shift1 : ArithShift  BitShiftNumberSource=Input port  BitShiftDirection=Right
      settings: InputPortMap=u0,p1
  xout : Outport  OutDataTypeStr=fixdt(1, 13, 0)
  yout : Outport  Port=2  OutDataTypeStr=fixdt(1, 13, 0)
  wires:
  idx/1 -> dynamic_shift/2, dynamic_shift1/2
  yin/1 -> compare/1, dynamic_shift1/1, YAdder/1, YSub/1
  xin/1 -> dynamic_shift/1, XSubtractor/1, XAdder/1
  YSub/1 -> MuxY/3
  YAdder/1 -> MuxY/1
  XAdder/1 -> MuxX/3
  XSubtractor/1 -> MuxX/1
  compare/1 -> MuxX/2, MuxY/2
  dynamic_shift1/1 -> XSubtractor/2, XAdder/2
  dynamic_shift/1 -> YAdder/2, YSub/2
  MuxY/1 -> yout/1
  MuxX/1 -> xout/1

== system gm_max_frequency_index/max_index_frequency/frequency_max/index_finder/for_each_instance32/Iteration2 ==
  xin : Inport  OutDataTypeStr=fixdt(1, 13, 0)  SampleTime=3.2e-05
  yin : Inport  Port=2  OutDataTypeStr=fixdt(1, 13, 0)  SampleTime=3.2e-05
  idx : Inport  Port=3  OutDataTypeStr=fixdt(0, 5, 0)  SampleTime=3.2e-05
  MuxX : Switch  Criteria=u2 ~= 0  Threshold=double(0)  OutDataTypeStr=fixdt(1, 13, 0)  SampleTime=3.2e-05
  MuxY : Switch  Criteria=u2 ~= 0  Threshold=double(0)  OutDataTypeStr=fixdt(1, 13, 0)  SampleTime=3.2e-05
  XAdder : Sum  OutDataTypeStr=fixdt(1, 13, 0)  SampleTime=3.2e-05
  XSubtractor : Sum  Inputs=+-  AccumDataTypeStr=fixdt(1, 13, 0)  OutDataTypeStr=fixdt(1, 13, 0)  SampleTime=3.2e-05
  YAdder : Sum  OutDataTypeStr=fixdt(1, 13, 0)  SampleTime=3.2e-05
  YSub : Sum  Inputs=+-  AccumDataTypeStr=fixdt(1, 13, 0)  OutDataTypeStr=fixdt(1, 13, 0)  SampleTime=3.2e-05
  compare : simulink/Logic and Bit Operations/Compare To Constant  relop=<  const=double(0)  OutDataTypeStr=boolean
  dynamic_shift : ArithShift  BitShiftNumberSource=Input port  BitShiftDirection=Right
      settings: InputPortMap=u0,p1
  dynamic_shift1 : ArithShift  BitShiftNumberSource=Input port  BitShiftDirection=Right
      settings: InputPortMap=u0,p1
  xout : Outport  OutDataTypeStr=fixdt(1, 13, 0)
  yout : Outport  Port=2  OutDataTypeStr=fixdt(1, 13, 0)
  wires:
  idx/1 -> dynamic_shift1/2, dynamic_shift/2
  yin/1 -> YSub/1, YAdder/1, dynamic_shift1/1, compare/1
  xin/1 -> XAdder/1, XSubtractor/1, dynamic_shift/1
  YSub/1 -> MuxY/3
  YAdder/1 -> MuxY/1
  XAdder/1 -> MuxX/3
  XSubtractor/1 -> MuxX/1
  compare/1 -> MuxY/2, MuxX/2
  dynamic_shift1/1 -> XAdder/2, XSubtractor/2
  dynamic_shift/1 -> YSub/2, YAdder/2
  MuxY/1 -> yout/1
  MuxX/1 -> xout/1

== system gm_max_frequency_index/max_index_frequency/frequency_max/index_finder/for_each_instance32/Iteration3 ==
  xin : Inport  OutDataTypeStr=fixdt(1, 13, 0)  SampleTime=3.2e-05
  yin : Inport  Port=2  OutDataTypeStr=fixdt(1, 13, 0)  SampleTime=3.2e-05
  idx : Inport  Port=3  OutDataTypeStr=fixdt(0, 5, 0)  SampleTime=3.2e-05
  MuxX : Switch  Criteria=u2 ~= 0  Threshold=double(0)  OutDataTypeStr=fixdt(1, 13, 0)  SampleTime=3.2e-05
  MuxY : Switch  Criteria=u2 ~= 0  Threshold=double(0)  OutDataTypeStr=fixdt(1, 13, 0)  SampleTime=3.2e-05
  XAdder : Sum  OutDataTypeStr=fixdt(1, 13, 0)  SampleTime=3.2e-05
  XSubtractor : Sum  Inputs=+-  AccumDataTypeStr=fixdt(1, 13, 0)  OutDataTypeStr=fixdt(1, 13, 0)  SampleTime=3.2e-05
  YAdder : Sum  OutDataTypeStr=fixdt(1, 13, 0)  SampleTime=3.2e-05
  YSub : Sum  Inputs=+-  AccumDataTypeStr=fixdt(1, 13, 0)  OutDataTypeStr=fixdt(1, 13, 0)  SampleTime=3.2e-05
  compare : simulink/Logic and Bit Operations/Compare To Constant  relop=<  const=double(0)  OutDataTypeStr=boolean
  dynamic_shift : ArithShift  BitShiftNumberSource=Input port  BitShiftDirection=Right
      settings: InputPortMap=u0,p1
  dynamic_shift1 : ArithShift  BitShiftNumberSource=Input port  BitShiftDirection=Right
      settings: InputPortMap=u0,p1
  xout : Outport  OutDataTypeStr=fixdt(1, 13, 0)
  yout : Outport  Port=2  OutDataTypeStr=fixdt(1, 13, 0)
  wires:
  idx/1 -> dynamic_shift1/2, dynamic_shift/2
  yin/1 -> YSub/1, YAdder/1, dynamic_shift1/1, compare/1
  xin/1 -> XAdder/1, XSubtractor/1, dynamic_shift/1
  YSub/1 -> MuxY/3
  YAdder/1 -> MuxY/1
  XAdder/1 -> MuxX/3
  XSubtractor/1 -> MuxX/1
  compare/1 -> MuxY/2, MuxX/2
  dynamic_shift1/1 -> XAdder/2, XSubtractor/2
  dynamic_shift/1 -> YSub/2, YAdder/2
  MuxY/1 -> yout/1
  MuxX/1 -> xout/1

== system gm_max_frequency_index/max_index_frequency/frequency_max/index_finder/for_each_instance32/Iteration4 ==
  xin : Inport  OutDataTypeStr=fixdt(1, 13, 0)  SampleTime=3.2e-05
  yin : Inport  Port=2  OutDataTypeStr=fixdt(1, 13, 0)  SampleTime=3.2e-05
  idx : Inport  Port=3  OutDataTypeStr=fixdt(0, 5, 0)  SampleTime=3.2e-05
  MuxX : Switch  Criteria=u2 ~= 0  Threshold=double(0)  OutDataTypeStr=fixdt(1, 13, 0)  SampleTime=3.2e-05
  MuxY : Switch  Criteria=u2 ~= 0  Threshold=double(0)  OutDataTypeStr=fixdt(1, 13, 0)  SampleTime=3.2e-05
  XAdder : Sum  OutDataTypeStr=fixdt(1, 13, 0)  SampleTime=3.2e-05
  XSubtractor : Sum  Inputs=+-  AccumDataTypeStr=fixdt(1, 13, 0)  OutDataTypeStr=fixdt(1, 13, 0)  SampleTime=3.2e-05
  YAdder : Sum  OutDataTypeStr=fixdt(1, 13, 0)  SampleTime=3.2e-05
  YSub : Sum  Inputs=+-  AccumDataTypeStr=fixdt(1, 13, 0)  OutDataTypeStr=fixdt(1, 13, 0)  SampleTime=3.2e-05
  compare : simulink/Logic and Bit Operations/Compare To Constant  relop=<  const=double(0)  OutDataTypeStr=boolean
  dynamic_shift : ArithShift  BitShiftNumberSource=Input port  BitShiftDirection=Right
      settings: InputPortMap=u0,p1
  dynamic_shift1 : ArithShift  BitShiftNumberSource=Input port  BitShiftDirection=Right
      settings: InputPortMap=u0,p1
  xout : Outport  OutDataTypeStr=fixdt(1, 13, 0)
  yout : Outport  Port=2  OutDataTypeStr=fixdt(1, 13, 0)
  wires:
  idx/1 -> dynamic_shift1/2, dynamic_shift/2
  yin/1 -> YSub/1, YAdder/1, dynamic_shift1/1, compare/1
  xin/1 -> XAdder/1, XSubtractor/1, dynamic_shift/1
  YSub/1 -> MuxY/3
  YAdder/1 -> MuxY/1
  XAdder/1 -> MuxX/3
  XSubtractor/1 -> MuxX/1
  compare/1 -> MuxY/2, MuxX/2
  dynamic_shift1/1 -> XAdder/2, XSubtractor/2
  dynamic_shift/1 -> YSub/2, YAdder/2
  MuxY/1 -> yout/1
  MuxX/1 -> xout/1

== system gm_max_frequency_index/max_index_frequency/frequency_max/index_finder/for_each_instance32/Iteration5 ==
  xin : Inport  OutDataTypeStr=fixdt(1, 13, 0)  SampleTime=3.2e-05
  yin : Inport  Port=2  OutDataTypeStr=fixdt(1, 13, 0)  SampleTime=3.2e-05
  idx : Inport  Port=3  OutDataTypeStr=fixdt(0, 5, 0)  SampleTime=3.2e-05
  MuxX : Switch  Criteria=u2 ~= 0  Threshold=double(0)  OutDataTypeStr=fixdt(1, 13, 0)  SampleTime=3.2e-05
  MuxY : Switch  Criteria=u2 ~= 0  Threshold=double(0)  OutDataTypeStr=fixdt(1, 13, 0)  SampleTime=3.2e-05
  XAdder : Sum  OutDataTypeStr=fixdt(1, 13, 0)  SampleTime=3.2e-05
  XSubtractor : Sum  Inputs=+-  AccumDataTypeStr=fixdt(1, 13, 0)  OutDataTypeStr=fixdt(1, 13, 0)  SampleTime=3.2e-05
  YAdder : Sum  OutDataTypeStr=fixdt(1, 13, 0)  SampleTime=3.2e-05
  YSub : Sum  Inputs=+-  AccumDataTypeStr=fixdt(1, 13, 0)  OutDataTypeStr=fixdt(1, 13, 0)  SampleTime=3.2e-05
  compare : simulink/Logic and Bit Operations/Compare To Constant  relop=<  const=double(0)  OutDataTypeStr=boolean
  dynamic_shift : ArithShift  BitShiftNumberSource=Input port  BitShiftDirection=Right
      settings: InputPortMap=u0,p1
  dynamic_shift1 : ArithShift  BitShiftNumberSource=Input port  BitShiftDirection=Right
      settings: InputPortMap=u0,p1
  xout : Outport  OutDataTypeStr=fixdt(1, 13, 0)
  yout : Outport  Port=2  OutDataTypeStr=fixdt(1, 13, 0)
  wires:
  idx/1 -> dynamic_shift1/2, dynamic_shift/2
  yin/1 -> YSub/1, YAdder/1, dynamic_shift1/1, compare/1
  xin/1 -> XAdder/1, XSubtractor/1, dynamic_shift/1
  YSub/1 -> MuxY/3
  YAdder/1 -> MuxY/1
  XAdder/1 -> MuxX/3
  XSubtractor/1 -> MuxX/1
  compare/1 -> MuxY/2, MuxX/2
  dynamic_shift1/1 -> XAdder/2, XSubtractor/2
  dynamic_shift/1 -> YSub/2, YAdder/2
  MuxY/1 -> yout/1
  MuxX/1 -> xout/1

== system gm_max_frequency_index/max_index_frequency/frequency_max/index_finder/for_each_instance32/Iteration6 ==
  xin : Inport  OutDataTypeStr=fixdt(1, 13, 0)  SampleTime=3.2e-05
  yin : Inport  Port=2  OutDataTypeStr=fixdt(1, 13, 0)  SampleTime=3.2e-05
  idx : Inport  Port=3  OutDataTypeStr=fixdt(0, 5, 0)  SampleTime=3.2e-05
  MuxX : Switch  Criteria=u2 ~= 0  Threshold=double(0)  OutDataTypeStr=fixdt(1, 13, 0)  SampleTime=3.2e-05
  MuxY : Switch  Criteria=u2 ~= 0  Threshold=double(0)  OutDataTypeStr=fixdt(1, 13, 0)  SampleTime=3.2e-05
  XAdder : Sum  OutDataTypeStr=fixdt(1, 13, 0)  SampleTime=3.2e-05
  XSubtractor : Sum  Inputs=+-  AccumDataTypeStr=fixdt(1, 13, 0)  OutDataTypeStr=fixdt(1, 13, 0)  SampleTime=3.2e-05
  YAdder : Sum  OutDataTypeStr=fixdt(1, 13, 0)  SampleTime=3.2e-05
  YSub : Sum  Inputs=+-  AccumDataTypeStr=fixdt(1, 13, 0)  OutDataTypeStr=fixdt(1, 13, 0)  SampleTime=3.2e-05
  compare : simulink/Logic and Bit Operations/Compare To Constant  relop=<  const=double(0)  OutDataTypeStr=boolean
  dynamic_shift : ArithShift  BitShiftNumberSource=Input port  BitShiftDirection=Right
      settings: InputPortMap=u0,p1
  dynamic_shift1 : ArithShift  BitShiftNumberSource=Input port  BitShiftDirection=Right
      settings: InputPortMap=u0,p1
  xout : Outport  OutDataTypeStr=fixdt(1, 13, 0)
  yout : Outport  Port=2  OutDataTypeStr=fixdt(1, 13, 0)
  wires:
  idx/1 -> dynamic_shift1/2, dynamic_shift/2
  yin/1 -> YSub/1, YAdder/1, dynamic_shift1/1, compare/1
  xin/1 -> XAdder/1, XSubtractor/1, dynamic_shift/1
  YSub/1 -> MuxY/3
  YAdder/1 -> MuxY/1
  XAdder/1 -> MuxX/3
  XSubtractor/1 -> MuxX/1
  compare/1 -> MuxY/2, MuxX/2
  dynamic_shift1/1 -> XAdder/2, XSubtractor/2
  dynamic_shift/1 -> YSub/2, YAdder/2
  MuxY/1 -> yout/1
  MuxX/1 -> xout/1

== system gm_max_frequency_index/max_index_frequency/frequency_max/index_finder/for_each_instance32/Iteration7 ==
  xin : Inport  OutDataTypeStr=fixdt(1, 13, 0)  SampleTime=3.2e-05
  yin : Inport  Port=2  OutDataTypeStr=fixdt(1, 13, 0)  SampleTime=3.2e-05
  idx : Inport  Port=3  OutDataTypeStr=fixdt(0, 5, 0)  SampleTime=3.2e-05
  MuxX : Switch  Criteria=u2 ~= 0  Threshold=double(0)  OutDataTypeStr=fixdt(1, 13, 0)  SampleTime=3.2e-05
  MuxY : Switch  Criteria=u2 ~= 0  Threshold=double(0)  OutDataTypeStr=fixdt(1, 13, 0)  SampleTime=3.2e-05
  XAdder : Sum  OutDataTypeStr=fixdt(1, 13, 0)  SampleTime=3.2e-05
  XSubtractor : Sum  Inputs=+-  AccumDataTypeStr=fixdt(1, 13, 0)  OutDataTypeStr=fixdt(1, 13, 0)  SampleTime=3.2e-05
  YAdder : Sum  OutDataTypeStr=fixdt(1, 13, 0)  SampleTime=3.2e-05
  YSub : Sum  Inputs=+-  AccumDataTypeStr=fixdt(1, 13, 0)  OutDataTypeStr=fixdt(1, 13, 0)  SampleTime=3.2e-05
  compare : simulink/Logic and Bit Operations/Compare To Constant  relop=<  const=double(0)  OutDataTypeStr=boolean
  dynamic_shift : ArithShift  BitShiftNumberSource=Input port  BitShiftDirection=Right
      settings: InputPortMap=u0,p1
  dynamic_shift1 : ArithShift  BitShiftNumberSource=Input port  BitShiftDirection=Right
      settings: InputPortMap=u0,p1
  xout : Outport  OutDataTypeStr=fixdt(1, 13, 0)
  yout : Outport  Port=2  OutDataTypeStr=fixdt(1, 13, 0)
  wires:
  idx/1 -> dynamic_shift1/2, dynamic_shift/2
  yin/1 -> YSub/1, YAdder/1, dynamic_shift1/1, compare/1
  xin/1 -> XAdder/1, XSubtractor/1, dynamic_shift/1
  YSub/1 -> MuxY/3
  YAdder/1 -> MuxY/1
  XAdder/1 -> MuxX/3
  XSubtractor/1 -> MuxX/1
  compare/1 -> MuxY/2, MuxX/2
  dynamic_shift1/1 -> XAdder/2, XSubtractor/2
  dynamic_shift/1 -> YSub/2, YAdder/2
  MuxY/1 -> yout/1
  MuxX/1 -> xout/1

== system gm_max_frequency_index/max_index_frequency/frequency_max/index_finder/for_each_instance32/Iteration8 ==
  xin : Inport  OutDataTypeStr=fixdt(1, 13, 0)  SampleTime=3.2e-05
  yin : Inport  Port=2  OutDataTypeStr=fixdt(1, 13, 0)  SampleTime=3.2e-05
  idx : Inport  Port=3  OutDataTypeStr=fixdt(0, 5, 0)  SampleTime=3.2e-05
  MuxX : Switch  Criteria=u2 ~= 0  Threshold=double(0)  OutDataTypeStr=fixdt(1, 13, 0)  SampleTime=3.2e-05
  MuxY : Switch  Criteria=u2 ~= 0  Threshold=double(0)  OutDataTypeStr=fixdt(1, 13, 0)  SampleTime=3.2e-05
  XAdder : Sum  OutDataTypeStr=fixdt(1, 13, 0)  SampleTime=3.2e-05
  XSubtractor : Sum  Inputs=+-  AccumDataTypeStr=fixdt(1, 13, 0)  OutDataTypeStr=fixdt(1, 13, 0)  SampleTime=3.2e-05
  YAdder : Sum  OutDataTypeStr=fixdt(1, 13, 0)  SampleTime=3.2e-05
  YSub : Sum  Inputs=+-  AccumDataTypeStr=fixdt(1, 13, 0)  OutDataTypeStr=fixdt(1, 13, 0)  SampleTime=3.2e-05
  compare : simulink/Logic and Bit Operations/Compare To Constant  relop=<  const=double(0)  OutDataTypeStr=boolean
  dynamic_shift : ArithShift  BitShiftNumberSource=Input port  BitShiftDirection=Right
      settings: InputPortMap=u0,p1
  dynamic_shift1 : ArithShift  BitShiftNumberSource=Input port  BitShiftDirection=Right
      settings: InputPortMap=u0,p1
  xout : Outport  OutDataTypeStr=fixdt(1, 13, 0)
  yout : Outport  Port=2  OutDataTypeStr=fixdt(1, 13, 0)
  wires:
  idx/1 -> dynamic_shift1/2, dynamic_shift/2
  yin/1 -> YSub/1, YAdder/1, dynamic_shift1/1, compare/1
  xin/1 -> XAdder/1, XSubtractor/1, dynamic_shift/1
  YSub/1 -> MuxY/3
  YAdder/1 -> MuxY/1
  XAdder/1 -> MuxX/3
  XSubtractor/1 -> MuxX/1
  compare/1 -> MuxY/2, MuxX/2
  dynamic_shift1/1 -> XAdder/2, XSubtractor/2
  dynamic_shift/1 -> YSub/2, YAdder/2
  MuxY/1 -> yout/1
  MuxX/1 -> xout/1

== system gm_max_frequency_index/max_index_frequency/frequency_max/index_finder/for_each_instance32/Iteration9 ==
  xin : Inport  OutDataTypeStr=fixdt(1, 13, 0)  SampleTime=3.2e-05
  yin : Inport  Port=2  OutDataTypeStr=fixdt(1, 13, 0)  SampleTime=3.2e-05
  idx : Inport  Port=3  OutDataTypeStr=fixdt(0, 5, 0)  SampleTime=3.2e-05
  MuxX : Switch  Criteria=u2 ~= 0  Threshold=double(0)  OutDataTypeStr=fixdt(1, 13, 0)  SampleTime=3.2e-05
  MuxY : Switch  Criteria=u2 ~= 0  Threshold=double(0)  OutDataTypeStr=fixdt(1, 13, 0)  SampleTime=3.2e-05
  XAdder : Sum  OutDataTypeStr=fixdt(1, 13, 0)  SampleTime=3.2e-05
  XSubtractor : Sum  Inputs=+-  AccumDataTypeStr=fixdt(1, 13, 0)  OutDataTypeStr=fixdt(1, 13, 0)  SampleTime=3.2e-05
  YAdder : Sum  OutDataTypeStr=fixdt(1, 13, 0)  SampleTime=3.2e-05
  YSub : Sum  Inputs=+-  AccumDataTypeStr=fixdt(1, 13, 0)  OutDataTypeStr=fixdt(1, 13, 0)  SampleTime=3.2e-05
  compare : simulink/Logic and Bit Operations/Compare To Constant  relop=<  const=double(0)  OutDataTypeStr=boolean
  dynamic_shift : ArithShift  BitShiftNumberSource=Input port  BitShiftDirection=Right
      settings: InputPortMap=u0,p1
  dynamic_shift1 : ArithShift  BitShiftNumberSource=Input port  BitShiftDirection=Right
      settings: InputPortMap=u0,p1
  xout : Outport  OutDataTypeStr=fixdt(1, 13, 0)
  yout : Outport  Port=2  OutDataTypeStr=fixdt(1, 13, 0)
  wires:
  idx/1 -> dynamic_shift1/2, dynamic_shift/2
  yin/1 -> YSub/1, YAdder/1, dynamic_shift1/1, compare/1
  xin/1 -> XAdder/1, XSubtractor/1, dynamic_shift/1
  YSub/1 -> MuxY/3
  YAdder/1 -> MuxY/1
  XAdder/1 -> MuxX/3
  XSubtractor/1 -> MuxX/1
  compare/1 -> MuxY/2, MuxX/2
  dynamic_shift1/1 -> XAdder/2, XSubtractor/2
  dynamic_shift/1 -> YSub/2, YAdder/2
  MuxY/1 -> yout/1
  MuxX/1 -> xout/1
